simulink model "notfullmod"  (R2014b)
settings: Solver=ode45  StartTime=0.0  StopTime=25.0  MaxStep=0.001  MinStep=0.0001  RelTol=1e-3
values from neighbouring files (symbols this model uses):
  ip = 20    [lab10.m]    (also in work.mat = 16; work2.mat = 16; work3.mat = 16; work4.mat = 16)
  Jsum = Jd+Jp+(Jm/(ip^2))    (= 0.01165)    [lab10.m]    (also in work.mat = 0.0126621875; work2.mat = 0.0126621875; work3.mat = 0.0126621875; work4.mat = 0.0126621875)
  K = Ky/(Ke*ip)    (= 1.256637)    [lab10.m]    (also in work.mat = 0.6545; work2.mat = 0.6545; work3.mat = 0.6545; work4.mat = 0.6545)
  Kalpha = 0.306647818047    [work3.mat]    (also in work4.mat)
  Kd = 1/R    (= 1.05263157895)    [lab10.m]    (also in work.mat = 1.33333333333; work2.mat = 1.33333333333; work3.mat = 1.33333333333; work4.mat = 1.33333333333)
  Ke = Un/Angular_velocity    (= 0.4376761149)    [lab10.m]    (also in work.mat = 0.716195569137; work2.mat = 0.716195569137; work3.mat = 0.716195569137; work4.mat = 0.716195569137)
  Kf = R/(Km*Ke*ip^2)    (= 0.0124806902045)    [lab10.m]    (also in work.mat = 0.008925; work2.mat = 0.008925; work3.mat = 0.008925; work4.mat = 0.008925)
  Ki = 0.292504570384    [work3.mat]    (also in work4.mat)
  Km = Mn/In    (= 0.434782608696)    [lab10.m]    (also in work.mat = 0.458333333333; work2.mat = 0.458333333333; work3.mat = 0.458333333333; work4.mat = 0.458333333333)
  Komega = 0.0954927425516    [work.mat]    (also in work2.mat; work3.mat = 0.190985485103; work4.mat = 0.190985485103)
  Ku = 0.133333333333    [work.mat]    (also in work2.mat; work3.mat = 0.266666666667; work4.mat = 0.266666666667)
  Ky = Un/Um    (= 11)    [lab10.m]    (also in work.mat = 7.5; work2.mat = 7.5; work3.mat = 7.5; work4.mat = 7.5)
  Tja = 0.007    [lab10.m]    (also in work.mat = 0.005; work2.mat = 0.005; work3.mat = 0.005; work4.mat = 0.005)
  Tm = (R*Jsum)/(Km*Ke)    (= 0.0581600163532)    [lab10.m]    (also in work.mat = 0.028930566; work2.mat = 0.028930566; work3.mat = 0.028930566; work4.mat = 0.028930566)
  Ty = 0.008    [lab10.m]    (also in work.mat = 0.006; work2.mat = 0.006; work3.mat = 0.006; work4.mat = 0.006)
settings Model: Creator=Игорь  LastModifiedBy=Игорь

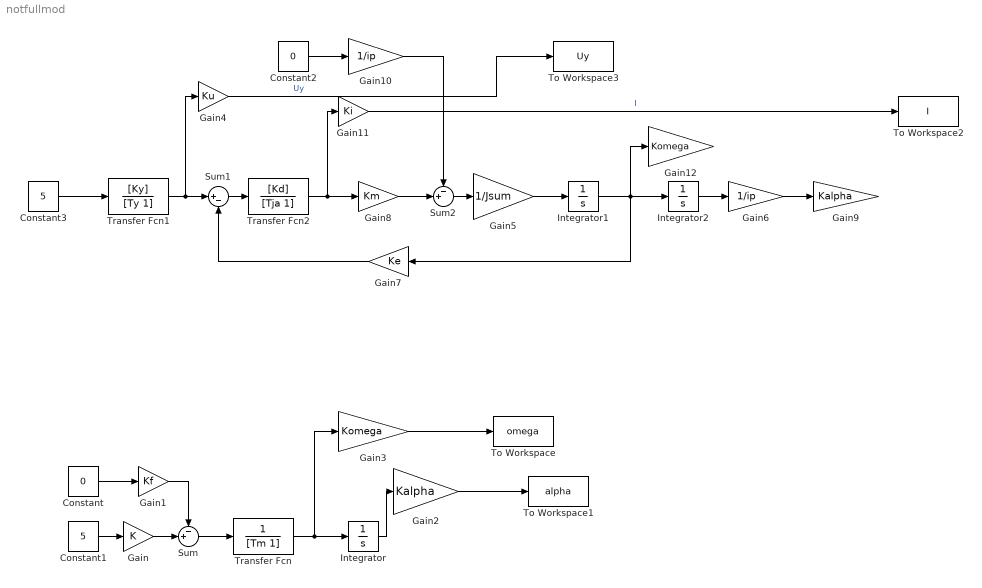
== system notfullmod ==
  Constant : Constant  Value=0
  Constant1 : Constant  Value=5
  Constant2 : Constant  Value=0
  Constant3 : Constant  Value=5
  Gain : Gain  Gain=K
  Gain1 : Gain  Gain=Kf
  Gain10 : Gain  Gain=1/ip
  Gain11 : Gain  Gain=Ki
  Gain12 : Gain  Gain=Komega
  Gain2 : Gain  Gain=Kalpha
  Gain3 : Gain  Gain=Komega
  Gain4 : Gain  Gain=Ku
  Gain5 : Gain  Gain=1/Jsum
  Gain6 : Gain  Gain=1/ip
  Gain7 : Gain  Gain=Ke
  Gain8 : Gain  Gain=Km
  Gain9 : Gain  Gain=Kalpha
  Integrator : Integrator
  Integrator1 : Integrator
  Integrator2 : Integrator
  Sum : Sum  Inputs=-+|
  Sum1 : Sum  Inputs=|+-
  Sum2 : Sum  Inputs=-+|
  To Workspace : ToWorkspace  VariableName=omega  SaveFormat=Timeseries  SampleTime=-1
  To Workspace1 : ToWorkspace  VariableName=alpha  SaveFormat=Timeseries  SampleTime=-1
  To Workspace2 : ToWorkspace  VariableName=I  SaveFormat=Timeseries  SampleTime=-1
  To Workspace3 : ToWorkspace  VariableName=Uy  SaveFormat=Timeseries  SampleTime=-1
  Transfer Fcn : TransferFcn  Denominator=[Tm 1]
  Transfer Fcn1 : TransferFcn  Numerator=[Ky]  Denominator=[Ty 1]
  Transfer Fcn2 : TransferFcn  Numerator=[Kd]  Denominator=[Tja 1]
  wires:
  Gain/1 -> Sum/2
  Constant1/1 -> Gain/1
  Constant/1 -> Gain1/1
  Gain1/1 -> Sum/1
  Sum/1 -> Transfer Fcn/1
  Transfer Fcn/1 -> Gain3/1, Integrator/1
  Integrator/1 -> Gain2/1
  Transfer Fcn1/1 -> Gain4/1, Sum1/1
  Sum1/1 -> Transfer Fcn2/1
  Gain7/1 -> Sum1/2
  Transfer Fcn2/1 -> Gain11/1, Gain8/1
  Gain8/1 -> Sum2/2
  Sum2/1 -> Gain5/1
  Gain5/1 -> Integrator1/1
  Integrator1/1 -> Gain7/1, Gain12/1, Integrator2/1
  Integrator2/1 -> Gain6/1
  Constant2/1 -> Gain10/1
  Gain10/1 -> Sum2/1
  Gain6/1 -> Gain9/1
  Constant3/1 -> Transfer Fcn1/1
  Gain4/1 -> To Workspace3/1  "Uy"
  Gain11/1 -> To Workspace2/1  "I"
  Gain3/1 -> To Workspace/1
  Gain2/1 -> To Workspace1/1
